simulink model "MSDRPrimaryLoop_LoadFollow"  (R2021b)
settings: Solver=VariableStepAuto  StartTime=0.0  StopTime=604900  MaxStep=1  MinStep=0.01  RelTol=1e-3
undefined symbols (not defined in the file): a_f, A_free_PHX, a_g, A_h_PHX, beta, beta_t, bubbleGeneratorArea, bubbleGeneratorDh, bubbleGeneratorElevation, bubbleGeneratorLength, bubbleGeneratorVolume, bubbleSaturationLevel, bubbleSeparatorArea, bubbleSeparatorDiameter, bubbleSeparatorDo, bubbleSeparatorLength, bubbleSeparatorSlope, bypassRatio, C0, coreFlowArea, coreFuelVolume, coreLowerPlenumArea, coreLowerPlenumHydraulicDiameter, coreLowerPlenumLength, coreLowerPlenumVolume, coreUpperPlenumArea, coreUpperPlenumHydraulicDiameter, coreUpperPlenumLength, coreUpperPlenumVolume, coreVolume, cpGraphite, dissolusionRatio, dMin, dScale, dsmConst, DXeG, Fiss_factor, fuelChannelHydrualicDiameter, fuelChannelLength, fuelDepositRatio, fuelFraction, fuelGraphiteArea, fuelGraphiteHeatTransferCoefficient, gamma0, gamma1, gamma2, generatorDsm, graphiteKDiff, graphiteUnitCellThickness, initialIodineConcentration, InitialXeMolarConcentration, InjectionRatio, injectionRatio, iodineDecayConstant, IodineDecayConstant, iodineYield, kGraphite, kScale, Lam, lam ... (+60)
libraries: fl_lib x268, nesl_utility x106, SimscapeFluids_lib x20, slpidlib x1
(part 6 of 12)

== system MSDRPrimaryLoop_LoadFollow/Pump/PumpIdeal/XenonCalcPump ==
  XeIn : Inport  OutDataTypeStr=double  Unit=kg/s
  GasRef : Inport  Port=2
  Absolute Reference (TL) : fl_lib/Thermal Liquid/Elements/Absolute Reference (TL)
      settings: SourceProductBaseCode=SS
  Demux : Demux  Outputs=2
  Gas : Subsystem
      settings: PortSchema="{\"entries\":[{\"content\":{\"sides\":[{\"content\":{\"connectorIds\":[\"In1\"]},\"type\":\"ConnectorPlacement.EquallySpacedRectSide\",\"uuid\":\"9457d014-8c8c-4ede-953a-dad1b8fcff2e\"},{\"content\":{\"connectorIds\":[\"Out1\"],\"side\":\"RIGHT\"},\"type\":\"ConnectorPlacement.EquallySpacedRectSide\",\"uuid\":\"6b13e550-1648-4662-a58b-f6f49b8dfc45\"},{\"content\":{\"connectorIds\":[\"Out2\",\"In2\"],\"side\":\"TOP\"},\"type\":\"ConnectorPlacement.EquallySpacedRectSide\",\"uuid\":\"73a4211d-b4c2-4f72-9c26-6ee46c1777bd\"},{\"content\":{\"connectorIds\":[\"In3\",\"In4\"],\"side\":\"BOTTOM\"},\"type\":\"ConnectorPlacement.EquallySpacedRectSide\",\"uuid\":\"ca62b0cd-46c8-418f-9a8b-9558726bf444\"}]},\"type\":\"ConnectorPlacement.EquallySpacedConnector\",\"uuid\":\"020f2da1-56fe-4a8a-8a2d-2f75d9123e14\"}],\"packageUris\":[\"http://schema.mathworks.com/mf0/Connector/R2020b\"],\"version\":\"1.0\"}"
  InterphaseTranfser : Subsystem
      settings: PortSchema="{\"entries\":[{\"content\":{\"sides\":[{\"content\":{\"connectorIds\":[\"In1\",\"In2\",\"In3\"]},\"type\":\"ConnectorPlacement.EquallySpacedRectSide\",\"uuid\":\"d6303689-138e-451a-a3c3-60d601b4795c\"},{\"content\":{\"connectorIds\":[\"Out1\"],\"side\":\"RIGHT\"},\"type\":\"ConnectorPlacement.EquallySpacedRectSide\",\"uuid\":\"e99266db-1ad9-4248-a3a9-dc80edd4cbf2\"},{\"content\":{\"connectorIds\":[\"LConn1\"],\"side\":\"TOP\"},\"type\":\"ConnectorPlacement.EquallySpacedRectSide\",\"uuid\":\"07679a3e-e535-452f-8d16-cac9376cf8bb\"}]},\"type\":\"ConnectorPlacement.EquallySpacedConnector\",\"uuid\":\"2a8870ca-366d-4312-85a0-e0a2095078d0\"}],\"packageUris\":[\"http://schema.mathworks.com/mf0/Connector/R2020b\"],\"version\":\"1.0\"}"
  Mux : Mux  Inputs=2
  PS Abs : fl_lib/Physical Signals/Nonlinear Operators/PS Abs
      settings: SourceProductBaseCode=SS  InternalSimscapePortConfiguration="{\"Bottom\":[],\"Left\":[{\"id\":\"I\",\"label\":\"\",\"type\":\"input\"}],\"Right\":[{\"id\":\"O\",\"label\":\"\",\"type\":\"output\"}],\"Top\":[]}"
  PS-Simulink Converter : nesl_utility/PS-Simulink Converter  PhysicalDomain=network_engine_domain  SubClassName=ps_output  LeftPortType=input  RightPortType=output  PseudoPeriodic=off  Frequencies=[]  Unit=inherit  AffineConversion=off
      settings: SourceProductBaseCode=PW,SS
  PS-Simulink Converter1 : nesl_utility/PS-Simulink Converter  PhysicalDomain=network_engine_domain  SubClassName=ps_output  LeftPortType=input  RightPortType=output  PseudoPeriodic=off  Frequencies=[]  Unit=inherit  AffineConversion=off
      settings: SourceProductBaseCode=PW,SS
  Pressure & Temperature Sensor (TL) : fl_lib/Thermal Liquid/Sensors/Pressure & Temperature Sensor (TL)
      settings: SourceProductBaseCode=SS  InternalSimscapePortConfiguration="{\"Bottom\":[],\"Left\":[{\"id\":\"A\",\"label\":\"A\",\"type\":\"foundation.thermal_liquid.thermal_liquid\"}],\"Right\":[{\"id\":\"B\",\"label\":\"B\",\"type\":\"foundation.thermal_liquid.thermal_liquid\"},{\"id\":\"P\",\"label\":\"P\",\"type\":\"output\"},{\"id\":\"T\",\"label\":\"T\",\"type\":\"output\"}],\"Top\":[]}"
  Salt : Subsystem
      settings: PortSchema="{\"entries\":[{\"content\":{\"sides\":[{\"content\":{\"connectorIds\":[\"In1\",\"In2\",\"In3\"]},\"type\":\"ConnectorPlacement.EquallySpacedRectSide\",\"uuid\":\"9457d014-8c8c-4ede-953a-dad1b8fcff2e\"},{\"content\":{\"connectorIds\":[\"Out1\"],\"side\":\"RIGHT\"},\"type\":\"ConnectorPlacement.EquallySpacedRectSide\",\"uuid\":\"6b13e550-1648-4662-a58b-f6f49b8dfc45\"},{\"content\":{\"connectorIds\":[\"In4\",\"In5\"],\"side\":\"TOP\"},\"type\":\"ConnectorPlacement.EquallySpacedRectSide\",\"uuid\":\"73a4211d-b4c2-4f72-9c26-6ee46c1777bd\"},{\"content\":{\"connectorIds\":[\"Out2\",\"In6\"],\"side\":\"BOTTOM\"},\"type\":\"ConnectorPlacement.EquallySpacedRectSide\",\"uuid\":\"ca62b0cd-46c8-418f-9a8b-9558726bf444\"}]},\"type\":\"ConnectorPlacement.EquallySpacedConnector\",\"uuid\":\"020f2da1-56fe-4a8a-8a2d-2f75d9123e14\"}],\"packageUris\":[\"http://schema.mathworks.com/mf0/Connector/R2020b\"],\"version\":\"1.0\"}"
  Volumetric Flow Rate Sensor (TL) : fl_lib/Thermal Liquid/Sensors/Volumetric Flow Rate Sensor (TL)
      settings: SourceProductBaseCode=SS  InternalSimscapePortConfiguration="{\"Bottom\":[],\"Left\":[{\"id\":\"A\",\"label\":\"A\",\"type\":\"foundation.thermal_liquid.thermal_liquid\"}],\"Right\":[{\"id\":\"B\",\"label\":\"B\",\"type\":\"foundation.thermal_liquid.thermal_liquid\"},{\"id\":\"V\",\"label\":\"V\",\"type\":\"output\"}],\"Top\":[]}"
  Inlet : PMIOPort  Side=Left
  Outlet : PMIOPort  Port=2  Side=Right
  XeOut : Outport
  wires:
  XeIn/1 -> Demux/1
  PS-Simulink Converter/1 -> Gas/4(VolumeRate), Salt/5(VolumeRate)
  GasRef/1 -> Gas/3(GasRef), InterphaseTranfser/2(GasRef), Salt/4(GasRef)
  Demux/1 -> Salt/1(XeLIn)
  [IodineSNDensity] -> Salt/2(IodineSNumberDensity)
  Demux/2 -> Gas/1(XeGIn)
  Salt/1(XeLOut) -> Mux/1
  Gas/1(XeGOut) -> Mux/2
  Mux/1 -> XeOut/1
  Salt/2(CxSalt) -> InterphaseTranfser/1(CxSalt)
  Gas/2(CxGas) -> InterphaseTranfser/3(CxGas)
  InterphaseTranfser/1(TranfserRate) -> Gas/2(Interphase), Salt/6(Interphase)
  PS-Simulink Converter1/1 -> Salt/3(T_f_ave)
  connections:
  Outlet/RConn1 -- Volumetric Flow Rate Sensor (TL)/RConn1 -- InterphaseTranfser/LConn1
  Volumetric Flow Rate Sensor (TL)/LConn1 -- Pressure & Temperature Sensor (TL)/LConn1 -- Inlet/RConn1
  Volumetric Flow Rate Sensor (TL)/RConn2 -- PS Abs/LConn1
  PS Abs/RConn1 -- PS-Simulink Converter/LConn1
  Pressure & Temperature Sensor (TL)/RConn1 -- Absolute Reference (TL)/LConn1
  Pressure & Temperature Sensor (TL)/RConn3 -- PS-Simulink Converter1/LConn1

== system MSDRPrimaryLoop_LoadFollow/Pump/PumpPysical/GasCalc ==
  GasIn : Inport
  Add : Sum  Inputs=+-
  GasExpansion : Subsystem  ReferencedSubsystem=GasExpansion
      settings: PortSchema="{\"entries\":[{\"content\":{\"sides\":[{\"content\":{\"connectorIds\":[\"LConn1\",\"In1\"]},\"type\":\"ConnectorPlacement.EquallySpacedRectSide\",\"uuid\":\"50c89675-cb8a-4964-af62-cb2014507b1d\"},{\"content\":{\"connectorIds\":[\"RConn1\",\"Out1\"],\"side\":\"RIGHT\"},\"type\":\"ConnectorPlacement.EquallySpacedRectSide\",\"uuid\":\"6b3adc78-0be5-4682-9da0-6fd41ffc4e71\"},{\"content\":{\"connectorIds\":[],\"side\":\"TOP\"},\"type\":\"ConnectorPlacement.EquallySpacedRectSide\",\"uuid\":\"5158b46f-a496-48e4-90d6-6c6dcc9e237b\"}]},\"type\":\"ConnectorPlacement.EquallySpacedConnector\",\"uuid\":\"7ff0188e-dc19-44a0-a8cf-bde33949414f\"}],\"packageUris\":[\"http://schema.mathworks.com/mf0/Connector/R2020b\"],\"version\":\"1.0\"}"
  Integrator : Integrator  InitialCondition=InjectionRatio*PumpVolume
  PS-Simulink Converter : nesl_utility/PS-Simulink Converter  PhysicalDomain=network_engine_domain  SubClassName=ps_output  LeftPortType=input  RightPortType=output  PseudoPeriodic=off  Frequencies=[]  Unit=inherit  AffineConversion=off
      settings: SourceProductBaseCode=PW,SS
  Product : Product
  VolumeToVoid : Gain  Gain=1/PumpVolume
  Ref1 : PMIOPort  Side=Left
  VolumeRate : PMIOPort  Port=2  Side=Left
  Ref2 : PMIOPort  Port=3  Side=Left
  GasOut : Outport
  wires:
  VolumeToVoid/1 -> GasExpansion/1, Add/2
  Integrator/1 -> VolumeToVoid/1
  GasIn/1 -> Add/1
  Add/1 -> Product/1
  Product/1 -> Integrator/1
  PS-Simulink Converter/1 -> Product/2
  GasExpansion/1 -> GasOut/1
  connections:
  PS-Simulink Converter/LConn1 -- VolumeRate/RConn1
  GasExpansion/LConn1 -- Ref1/RConn1
  GasExpansion/RConn1 -- Ref2/RConn1

== system MSDRPrimaryLoop_LoadFollow/Pump/PumpPysical/PumpPhysics&Control ==
  note: Pump capacity is linearly scaled to 3 times of the deisgn, as only one loop is modeled.
  GasRef : Inport
  2PModification : Subsystem  ReferencedSubsystem=TwoPhaseModification
      settings: PortSchema="{\"entries\":[{\"content\":{\"sides\":[{\"content\":{\"connectorIds\":[\"LConn1\"]},\"type\":\"ConnectorPlacement.EquallySpacedRectSide\",\"uuid\":\"7546b4b7-b669-49c8-8f27-f696391ea3ad\"},{\"content\":{\"connectorIds\":[\"RConn1\"],\"side\":\"RIGHT\"},\"type\":\"ConnectorPlacement.EquallySpacedRectSide\",\"uuid\":\"0e6176f2-177c-4327-bcfa-9a190fe9083f\"},{\"content\":{\"connectorIds\":[\"RConn2\"],\"side\":\"TOP\"},\"type\":\"ConnectorPlacement.EquallySpacedRectSide\",\"uuid\":\"16faf74c-4635-4009-a5b3-33dd03b625c6\"},{\"content\":{\"connectorIds\":[\"LConn2\",\"In1\"],\"side\":\"BOTTOM\"},\"type\":\"ConnectorPlacement.EquallySpacedRectSide\",\"uuid\":\"2081d73b-bb08-4ad9-b5c8-e48a4e9c4e20\"}]},\"type\":\"ConnectorPlacement.EquallySpacedConnector\",\"uuid\":\"243e4075-206b-4747-a8bc-b8f10d9a577f\"}],\"packageUris\":[\"http://schema.mathworks.com/mf0/Connector/R2020b\"],\"version\":\"1.0\"}"
  Centrifugal Pump (TL) : SimscapeFluids_lib/Thermal Liquid/Pumps & Motors/Centrifugal Pump (TL)  pump_parameterization=fluids.thermal_liquid.pumps_motors.enum.CentrifugalPumpParameterization.Nominal  capacity_ref_nominal=v_dot m^3/s  head_ref_nominal=45.7200 m  power_ref_nominal=0.85 kW  head_ref_max=70 m  capacity_ref_max=v_dot*2 m^3/s  omega_ref_analytic=2500 rpm  flow_rate_1D_TLU=[16.67, 30, 40, 53.33, 66.67, 83.33] lpm  head_1D_TLU=[50, 47.5, 45, 40, 35, 25] m  power_1D_TLU=[.6, .75, .85, .93, .98, .99] kW  omega_ref_1D=3500 rpm  rho_ref_1D=998.21 kg/m^3  flow_rate_2D_TLU=[16.67, 23.33, 30, 40, 53.33, 60] lpm  omega_2D_TLU=[2450, 2800, 3150, 3500] rpm  head_2D_TLU=[25, 32.7, 42.5, 50; 24, 31.7, 41, 49; 22.7, 30.5, 39, 47.5; 20, 28, 36, 45; 15.7, 24, 32, 40; 12.5, 21, 29.5, 37.5] m  power_2D_TLU=[.28, .38, .5, .6; .31, .41, .55, .68; .33, .44, .6, .75; .36, .48, .65, .83; .38, .53, .72, .93; .39, .55, .75, .97] kW  rho_ref_2D=998.21 kg/m^3  diameter_ratio=1  mech_orientation=fluids.thermal_liquid.pumps_motors.enum.CentrifugalPumpMechOrientation.Positive  area=0.25*pi*Pipe1Diameter^2*3 m^2
      settings: SourceProductBaseCode=SH  LogSimulationData=on  InternalSimscapePortConfiguration="{\"Bottom\":[],\"Left\":[{\"id\":\"A\",\"label\":\"A\",\"type\":\"foundation.thermal_liquid.thermal_liquid\"},{\"id\":\"B\",\"label\":\"B\",\"type\":\"foundation.thermal_liquid.thermal_liquid\"}],\"Right\":[{\"id\":\"R\",\"label\":\"R\",\"type\":\"foundation.mechanical.rotational.rotational\"},{\"id\":\"C\",\"label\":\"C\",\"type\":\"foundation.mechanical.rotational.rotational\"}],\"Top\":[]}"
  Ideal Angular Velocity Source : fl_lib/Mechanical/Mechanical Sources/Ideal Angular Velocity Source
  Mechanical Rotational Reference1 : fl_lib/Mechanical/Rotational Elements/Mechanical Rotational Reference
  Mechanical Rotational Reference2 : fl_lib/Mechanical/Rotational Elements/Mechanical Rotational Reference
  PS Abs : fl_lib/Physical Signals/Nonlinear Operators/PS Abs
      settings: SourceProductBaseCode=SS  InternalSimscapePortConfiguration="{\"Bottom\":[],\"Left\":[{\"id\":\"I\",\"label\":\"\",\"type\":\"input\"}],\"Right\":[{\"id\":\"O\",\"label\":\"\",\"type\":\"output\"}],\"Top\":[]}"
  Pump Drive Control : Subsystem
      settings: PortSchema="{\"entries\":[{\"content\":{\"sides\":[{\"content\":{\"connectorIds\":[\"LConn1\"]},\"type\":\"ConnectorPlacement.EquallySpacedRectSide\",\"uuid\":\"e4f8502b-306b-4a14-917e-1e63d742dab0\"},{\"content\":{\"connectorIds\":[\"RConn1\"],\"side\":\"RIGHT\"},\"type\":\"ConnectorPlacement.EquallySpacedRectSide\",\"uuid\":\"711ed699-17a5-44fb-968d-5c6132c14151\"},{\"content\":{\"connectorIds\":[\"LConn2\"],\"side\":\"TOP\"},\"type\":\"ConnectorPlacement.EquallySpacedRectSide\",\"uuid\":\"4e78022b-898e-4d83-b0bd-b0ef3bc93923\"},{\"content\":{\"connectorIds\":[],\"side\":\"BOTTOM\"},\"type\":\"ConnectorPlacement.EquallySpacedRectSide\",\"uuid\":\"a73c464e-7373-4480-b96b-ebe915c98bdf\"}]},\"type\":\"ConnectorPlacement.EquallySpacedConnector\",\"uuid\":\"08f647c4-2347-4031-ac16-01138a2dbc22\"}],\"packageUris\":[\"http://schema.mathworks.com/mf0/Connector/R2020b\"],\"version\":\"1.0\"}"
  PumpBowl : fl_lib/Thermal Liquid/Elements/Reservoir (TL)  pressure_spec=foundation.enum.pressure_spec.specified  reservoir_pressure=P0 Pa  reservoir_temperature=700 K  area=0.01 m^2
      settings: SourceProductBaseCode=SS  LogSimulationData=on
  Volumetric Flow Rate Sensor (TL) : fl_lib/Thermal Liquid/Sensors/Volumetric Flow Rate Sensor (TL)
      settings: SourceProductBaseCode=SS  InternalSimscapePortConfiguration="{\"Bottom\":[],\"Left\":[{\"id\":\"A\",\"label\":\"A\",\"type\":\"foundation.thermal_liquid.thermal_liquid\"}],\"Right\":[{\"id\":\"B\",\"label\":\"B\",\"type\":\"foundation.thermal_liquid.thermal_liquid\"},{\"id\":\"V\",\"label\":\"V\",\"type\":\"output\"}],\"Top\":[]}"
  Inlet : PMIOPort  Side=Left
  Outlet : PMIOPort  Port=2  Side=Right
  VolumeRate : PMIOPort  Port=3  Side=Right
  wires:
  GasRef/1 -> 2PModification/1
  connections:
  Ideal Angular Velocity Source/RConn1 -- Pump Drive Control/LConn1
  Centrifugal Pump (TL)/LConn1 -- 2PModification/LConn2 -- PumpBowl/LConn1 -- Inlet/RConn1 -- Pump Drive Control/RConn1
  Centrifugal Pump (TL)/RConn1 -- Ideal Angular Velocity Source/LConn1
  Centrifugal Pump (TL)/RConn2 -- Mechanical Rotational Reference2/LConn1
  Ideal Angular Velocity Source/RConn2 -- Mechanical Rotational Reference1/LConn1
  Volumetric Flow Rate Sensor (TL)/RConn2 -- PS Abs/LConn1
  Centrifugal Pump (TL)/LConn2 -- Volumetric Flow Rate Sensor (TL)/LConn1
  PS Abs/RConn1 -- VolumeRate/RConn1 -- Pump Drive Control/LConn2
  Volumetric Flow Rate Sensor (TL)/RConn1 -- 2PModification/RConn2 -- 2PModification/LConn1
  2PModification/RConn1 -- Outlet/RConn1

== system MSDRPrimaryLoop_LoadFollow/Pump/PumpPysical/XenonCalc ==
  XeIn : Inport
  Add : Sum  Inputs=|+--
  Decay : Gain  Gain=XeDecayConstant
  MassToConc : Gain  Gain=1/PumpVolume
  PS-Simulink Converter : nesl_utility/PS-Simulink Converter  PhysicalDomain=network_engine_domain  SubClassName=ps_output  LeftPortType=input  RightPortType=output  PseudoPeriodic=off  Frequencies=[]  Unit=inherit  AffineConversion=off
      settings: SourceProductBaseCode=PW,SS
  Product : Product
  TotalMass : Integrator  InitialCondition=InitialXeMolarConcentration*PumpVolume*0.135
  VolumeRate : PMIOPort  Side=Left
  XeOut : Outport
  wires:
  Add/1 -> TotalMass/1
  XeIn/1 -> Add/1
  Product/1 -> Add/3, XeOut/1
  TotalMass/1 -> Decay/1, MassToConc/1
  PS-Simulink Converter/1 -> Product/1
  MassToConc/1 -> Product/2
  Decay/1 -> Add/2
  connections:
  VolumeRate/RConn1 -- PS-Simulink Converter/LConn1

== system MSDRPrimaryLoop_LoadFollow/Reactor/CoreTH&Inerti/Core ==
  XeIn : Inport
  GasIn : Inport  Port=2
  IodineSNumberDensity : Inport  Port=3
  NeutronFraction : Inport  Port=4
  DecayFraction : Inport  Port=5
  CoreTH : Subsystem  mask{N_nodes=4, FuelDepositRatio=fuelDepositRatio, k_graphite=kGraphite, cp_graphite=cpGraphite, rho_graphite=rhoGraphite, UnitCellGraphiteThickness=graphiteUnitCellThickness, h_fg=fuelGraphiteHeatTransferCoefficient, T0=T0, P0=P0}
      mask prompts: N_nodes "Number Of Nodes"; k_graphite "Graphite Thermal Conductivity"; cp_graphite "Graphite Specific Thermal Capacity"; rho_graphite "Graphite Density"; UnitCellGraphiteThickness "Unit Cell Graphite Thickness"; h_fg "Fuel Graphite Heat Transfer Coefficient"; T0 "Initial Temperature"; P0 "Initial Pressure"
      settings: PortSchema="{\"entries\":[{\"content\":{\"sides\":[{\"content\":{\"connectorIds\":[\"LConn1\",\"LConn2\",\"LConn3\"]},\"type\":\"ConnectorPlacement.EquallySpacedRectSide\",\"uuid\":\"1c20b62e-1aca-4cc3-9434-4d9ffc0779e4\"},{\"content\":{\"connectorIds\":[\"Out1\",\"RConn1\"],\"side\":\"RIGHT\"},\"type\":\"ConnectorPlacement.EquallySpacedRectSide\",\"uuid\":\"cbe92cdf-09f7-4580-a6a7-168080192112\"},{\"content\":{\"connectorIds\":[\"In1\",\"In2\"],\"side\":\"TOP\"},\"type\":\"ConnectorPlacement.EquallySpacedRectSide\",\"uuid\":\"70a4d7aa-1432-4349-89f0-42a0194e580f\"},{\"content\":{\"connectorIds\":[\"In3\"],\"side\":\"BOTTOM\"},\"type\":\"ConnectorPlacement.EquallySpacedRectSide\",\"uuid\":\"7c92aed1-92dd-461a-937a-8dd840527e94\"}]},\"type\":\"ConnectorPlacement.EquallySpacedConnector\",\"uuid\":\"1a67b279-14f5-41a4-8cd2-abe76a0f00c3\"}],\"packageUris\":[\"http://schema.mathworks.com/mf0/Connector/R2020b\"],\"version\":\"1.0\"}"
  CoreXenonCalc : Subsystem
      settings: PortSchema="{\"entries\":[{\"content\":{\"sides\":[{\"content\":{\"connectorIds\":[\"In1\",\"LConn1\"]},\"type\":\"ConnectorPlacement.EquallySpacedRectSide\",\"uuid\":\"82f8e7e7-fd89-4597-952e-64db268d0190\"},{\"content\":{\"connectorIds\":[\"Out1\",\"Out2\",\"RConn1\"],\"side\":\"RIGHT\"},\"type\":\"ConnectorPlacement.EquallySpacedRectSide\",\"uuid\":\"4b3edad1-18f8-43fa-96ee-a24bb3384b59\"},{\"content\":{\"connectorIds\":[\"In2\",\"In3\",\"In4\"],\"side\":\"TOP\"},\"type\":\"ConnectorPlacement.EquallySpacedRectSide\",\"uuid\":\"43d4f51d-f841-40d6-804e-7f238a90dabe\"},{\"content\":{\"connectorIds\":[\"In5\",\"In6\"],\"side\":\"BOTTOM\"},\"type\":\"ConnectorPlacement.EquallySpacedRectSide\",\"uuid\":\"350f2274-4108-4e6e-a637-0ae7118de3f0\"}]},\"type\":\"ConnectorPlacement.EquallySpacedConnector\",\"uuid\":\"d7e795ea-9d5d-4a8c-83ab-dab42197cc2f\"}],\"packageUris\":[\"http://schema.mathworks.com/mf0/Connector/R2020b\"],\"version\":\"1.0\"}"
  Delay One Step : Delay  DelayLength=1  InitialCondition=T0
  PLossFunc : Subsystem
      settings: PortSchema="{\"entries\":[{\"content\":{\"sides\":[{\"content\":{\"connectorIds\":[\"Out1\",\"LConn1\"]},\"type\":\"ConnectorPlacement.EquallySpacedRectSide\",\"uuid\":\"95ca4545-c473-4e31-844b-c43557042c16\"},{\"content\":{\"connectorIds\":[\"RConn1\"],\"side\":\"RIGHT\"},\"type\":\"ConnectorPlacement.EquallySpacedRectSide\",\"uuid\":\"f9304c30-8684-4a05-a34b-3121610e628d\"},{\"content\":{\"connectorIds\":[],\"side\":\"TOP\"},\"type\":\"ConnectorPlacement.EquallySpacedRectSide\",\"uuid\":\"64c7a4d8-8539-4303-ae81-4015bd1451af\"}]},\"type\":\"ConnectorPlacement.EquallySpacedConnector\",\"uuid\":\"40c12b2f-fb9d-4a19-b6f1-e93ae1fd4d68\"}],\"packageUris\":[\"http://schema.mathworks.com/mf0/Connector/R2020b\"],\"version\":\"1.0\"}"
  SolubilityReduction : Subsystem
      settings: PortSchema="{\"entries\":[{\"content\":{\"sides\":[{\"content\":{\"connectorIds\":[\"In1\",\"In2\"]},\"type\":\"ConnectorPlacement.EquallySpacedRectSide\",\"uuid\":\"faacc406-4069-496b-af99-41d2aed9dfc2\"},{\"content\":{\"connectorIds\":[\"Out1\",\"Out2\",\"Out3\"],\"side\":\"RIGHT\"},\"type\":\"ConnectorPlacement.EquallySpacedRectSide\",\"uuid\":\"94f1539c-5515-4bd6-bffb-3a5caf43f7b6\"},{\"content\":{\"connectorIds\":[],\"side\":\"TOP\"},\"type\":\"ConnectorPlacement.EquallySpacedRectSide\",\"uuid\":\"d17dce47-2058-4206-8706-4dc771d04045\"},{\"content\":{\"connectorIds\":[\"Out4\"],\"side\":\"BOTTOM\"},\"type\":\"ConnectorPlacement.EquallySpacedRectSide\",\"uuid\":\"97529780-84fa-4776-a404-e5a3e7258a40\"}]},\"type\":\"ConnectorPlacement.EquallySpacedConnector\",\"uuid\":\"1ce9374c-8c3e-43ec-9da7-5b483b5e3d48\"}],\"packageUris\":[\"http://schema.mathworks.com/mf0/Connector/R2020b\"],\"version\":\"1.0\"}"
  Subsystem : Subsystem
  Subsystem1 : Subsystem
      settings: PortSchema="{\"entries\":[{\"content\":{\"sides\":[{\"content\":{\"connectorIds\":[\"In1\",\"In2\"]},\"type\":\"ConnectorPlacement.EquallySpacedRectSide\",\"uuid\":\"2a068eb5-92e4-43e3-b748-0f561ebb2f0e\"},{\"content\":{\"connectorIds\":[\"Out1\",\"Out2\"],\"side\":\"RIGHT\"},\"type\":\"ConnectorPlacement.EquallySpacedRectSide\",\"uuid\":\"d07e14f8-d0ba-4d92-9a78-613216e777c8\"},{\"content\":{\"connectorIds\":[\"LConn1\",\"LConn2\",\"Out3\",\"LConn3\"],\"side\":\"TOP\"},\"type\":\"ConnectorPlacement.EquallySpacedRectSide\",\"uuid\":\"40c9f9fd-9b75-4721-9a62-c538b0ea8b4c\"}]},\"type\":\"ConnectorPlacement.EquallySpacedConnector\",\"uuid\":\"1283fec4-e55b-4051-bba7-bc8dde4dc12d\"}],\"packageUris\":[\"http://schema.mathworks.com/mf0/Connector/R2020b\"],\"version\":\"1.0\"}"
  Subsystem2 : Subsystem  Variant=on  VariantControlMode=label  VariantControl=Choice  LabelModeActiveChoice=Constant
      settings: PortSchema="{\"entries\":[{\"content\":{\"sides\":[{\"content\":{\"connectorIds\":[\"In1\",\"In2\",\"In3\"]},\"type\":\"ConnectorPlacement.EquallySpacedRectSide\",\"uuid\":\"cfe1ce7c-1611-431e-9412-2b3caba343b3\"},{\"content\":{\"connectorIds\":[\"Out1\",\"Out2\"],\"side\":\"RIGHT\"},\"type\":\"ConnectorPlacement.EquallySpacedRectSide\",\"uuid\":\"0c689a27-e89a-4b17-8ea0-ad5769387ae3\"},{\"content\":{\"connectorIds\":[\"In4\"],\"side\":\"TOP\"},\"type\":\"ConnectorPlacement.EquallySpacedRectSide\",\"uuid\":\"a650924a-5c90-44bf-97de-77f017d49b56\"},{\"content\":{\"connectorIds\":[\"In5\"],\"side\":\"BOTTOM\"},\"type\":\"ConnectorPlacement.EquallySpacedRectSide\",\"uuid\":\"af91b143-b368-4d0c-8cc7-2ed084fb2df7\"}]},\"type\":\"ConnectorPlacement.EquallySpacedConnector\",\"uuid\":\"a7e506ef-3f33-4307-859c-c22ba4b969e5\"}],\"packageUris\":[\"http://schema.mathworks.com/mf0/Connector/R2020b\"],\"version\":\"1.0\"}"
  Volumetric Flow Rate Sensor (TL) : fl_lib/Thermal Liquid/Sensors/Volumetric Flow Rate Sensor (TL)
      settings: SourceProductBaseCode=SS  InternalSimscapePortConfiguration="{\"Bottom\":[],\"Left\":[{\"id\":\"A\",\"label\":\"A\",\"type\":\"foundation.thermal_liquid.thermal_liquid\"}],\"Right\":[{\"id\":\"B\",\"label\":\"B\",\"type\":\"foundation.thermal_liquid.thermal_liquid\"},{\"id\":\"V\",\"label\":\"V\",\"type\":\"output\"}],\"Top\":[]}"
  Inlet : PMIOPort  Side=Left
  InletSideHeatTranfser : PMIOPort  Port=2  Side=Left
  Outlet : PMIOPort  Port=3  Side=Right
  " Outlet Side Heat Transfer" : PMIOPort  Port=4  Side=Right
  XeOut : Outport
  GasOut : Outport  Port=2
  "TotalXeCrossSection, [cm^2]" : Outport  Port=3
  Temperatures : Outport  Port=4
  wires:
  NeutronFraction/1 -> CoreTH/2(NeutronFraction), CoreXenonCalc/4(NeutronFraction)
  CoreTH/1(Temperatures) -> Temperatures/1, Subsystem/1(Temperatures)
  XeIn/1 -> SolubilityReduction/1(XeIn)
  Delay One Step/1 -> CoreXenonCalc/3(T_f_ave), Subsystem2/4(Temperature)
  CoreXenonCalc/2("TotalXeCrossSection, [cm^2]") -> "TotalXeCrossSection, [cm^2]"/1
  Subsystem/1(T_f_ave) -> Delay One Step/1
  IodineSNumberDensity/1 -> CoreXenonCalc/2(IodineSNumberDensity)
  SolubilityReduction/1(XeOut) -> CoreXenonCalc/1(XeIn)
  GasIn/1 -> SolubilityReduction/2(GasIn)
  DecayFraction/1 -> CoreTH/1(DecayFraction)
  Subsystem1/3(GasRefOut) -> CoreTH/3(GasRef), CoreXenonCalc/6(GasRef)
  SolubilityReduction/2(GasOut) -> Subsystem1/1(GasIn)
  SolubilityReduction/3(AbsorbedGas) -> Subsystem1/2(Absorbed)
  PLossFunc/1(PLoss) -> CoreXenonCalc/5(PLoss)
  CoreXenonCalc/1(XeOut) -> Subsystem2/1(XeIn)
  Subsystem1/1(GasOut) -> Subsystem2/2(GasIn)
  Subsystem1/2(AbsorbedOut) -> Subsystem2/3(AbsorbedOut)
  SolubilityReduction/4(ModeSwitch) -> Subsystem2/5(ModeSwitch)
  Subsystem2/1(GasOut) -> GasOut/1
  Subsystem2/2(XeOut) -> XeOut/1
  connections:
  Volumetric Flow Rate Sensor (TL)/LConn1 -- PLossFunc/LConn1 -- Subsystem1/LConn1 -- Inlet/RConn1
  Volumetric Flow Rate Sensor (TL)/RConn1 -- CoreXenonCalc/LConn1
  CoreXenonCalc/RConn1 -- CoreTH/LConn1
  CoreTH/RConn1 -- Outlet/RConn1 -- PLossFunc/RConn1 -- Subsystem1/LConn3
  Volumetric Flow Rate Sensor (TL)/RConn2 -- Subsystem1/LConn2
  CoreTH/LConn2 -- InletSideHeatTranfser/RConn1
  CoreTH/LConn3 -- " Outlet Side Heat Transfer"/RConn1

== system MSDRPrimaryLoop_LoadFollow/Reactor/CoreTH&Inerti/LowerPlenum ==
  XeIn : Inport
  GasIn : Inport  Port=2
  Add : Sum  Inputs=|++
  Delay One Step : Delay  DelayLength=1
  Gain : Gain  Gain=0.5
  GasCalc : Subsystem  mask{Volume=Volume}
      settings: PortSchema="{\"entries\":[{\"content\":{\"sides\":[{\"content\":{\"connectorIds\":[\"In1\"]},\"type\":\"ConnectorPlacement.EquallySpacedRectSide\",\"uuid\":\"a8e1ce06-71c9-462d-8d5c-7a3e078b5544\"},{\"content\":{\"connectorIds\":[\"Out1\"],\"side\":\"RIGHT\"},\"type\":\"ConnectorPlacement.EquallySpacedRectSide\",\"uuid\":\"2c63a1ce-15e2-4b17-a432-f9f40781bd58\"},{\"content\":{\"connectorIds\":[\"LConn1\",\"LConn2\",\"LConn3\"],\"side\":\"TOP\"},\"type\":\"ConnectorPlacement.EquallySpacedRectSide\",\"uuid\":\"abc20e07-15eb-475f-be7f-cc96378523a1\"},{\"content\":{\"connectorIds\":[],\"side\":\"BOTTOM\"},\"type\":\"ConnectorPlacement.EquallySpacedRectSide\",\"uuid\":\"ab58f362-f4c2-4e86-bda0-802426066295\"}]},\"type\":\"ConnectorPlacement.EquallySpacedConnector\",\"uuid\":\"b54d49a9-048b-4912-bf18-92a7ef5e8aff\"}],\"packageUris\":[\"http://schema.mathworks.com/mf0/Connector/R2020b\"],\"version\":\"1.0\"}"
  LowerPlenum : Subsystem
      settings: PortSchema="{\"entries\":[{\"content\":{\"sides\":[{\"content\":{\"connectorIds\":[\"LConn1\",\"In1\"]},\"type\":\"ConnectorPlacement.EquallySpacedRectSide\",\"uuid\":\"0f255306-ec83-4423-ac41-a2708bd1ec44\"},{\"content\":{\"connectorIds\":[\"RConn1\",\"RConn2\"],\"side\":\"RIGHT\"},\"type\":\"ConnectorPlacement.EquallySpacedRectSide\",\"uuid\":\"650fb4ea-7b32-4c45-8538-9785d9ca64bf\"},{\"content\":{\"connectorIds\":[],\"side\":\"TOP\"},\"type\":\"ConnectorPlacement.EquallySpacedRectSide\",\"uuid\":\"434d3568-54a4-4787-a287-69f15ef478cb\"},{\"content\":{\"connectorIds\":[\"RConn3\"],\"side\":\"BOTTOM\"},\"type\":\"ConnectorPlacement.EquallySpacedRectSide\",\"uuid\":\"5b0b510d-1175-4508-bbe9-65b563e28484\"}]},\"type\":\"ConnectorPlacement.EquallySpacedConnector\",\"uuid\":\"b18d9c84-3d71-444b-a89d-79c3dc70d4d9\"}],\"packageUris\":[\"http://schema.mathworks.com/mf0/Connector/R2020b\"],\"version\":\"1.0\"}"
  PLossFunc : Subsystem
      settings: PortSchema="{\"entries\":[{\"content\":{\"sides\":[{\"content\":{\"connectorIds\":[\"Out1\",\"LConn1\"]},\"type\":\"ConnectorPlacement.EquallySpacedRectSide\",\"uuid\":\"95ca4545-c473-4e31-844b-c43557042c16\"},{\"content\":{\"connectorIds\":[\"RConn1\"],\"side\":\"RIGHT\"},\"type\":\"ConnectorPlacement.EquallySpacedRectSide\",\"uuid\":\"f9304c30-8684-4a05-a34b-3121610e628d\"},{\"content\":{\"connectorIds\":[],\"side\":\"TOP\"},\"type\":\"ConnectorPlacement.EquallySpacedRectSide\",\"uuid\":\"64c7a4d8-8539-4303-ae81-4015bd1451af\"}]},\"type\":\"ConnectorPlacement.EquallySpacedConnector\",\"uuid\":\"40c12b2f-fb9d-4a19-b6f1-e93ae1fd4d68\"}],\"packageUris\":[\"http://schema.mathworks.com/mf0/Connector/R2020b\"],\"version\":\"1.0\"}"
  XenonCalc : Subsystem  mask{Volume=Volume, Area=Area, Length=Length, Dh=Dh, Elevation=Elevation}
      mask prompts: Dh "Hydraulic Diameter"
      settings: PortSchema="{\"entries\":[{\"content\":{\"sides\":[{\"content\":{\"connectorIds\":[\"LConn1\",\"In1\"]},\"type\":\"ConnectorPlacement.EquallySpacedRectSide\",\"uuid\":\"82f8e7e7-fd89-4597-952e-64db268d0190\"},{\"content\":{\"connectorIds\":[\"RConn1\",\"Out1\"],\"side\":\"RIGHT\"},\"type\":\"ConnectorPlacement.EquallySpacedRectSide\",\"uuid\":\"4b3edad1-18f8-43fa-96ee-a24bb3384b59\"},{\"content\":{\"connectorIds\":[\"In2\"],\"side\":\"TOP\"},\"type\":\"ConnectorPlacement.EquallySpacedRectSide\",\"uuid\":\"43d4f51d-f841-40d6-804e-7f238a90dabe\"},{\"content\":{\"connectorIds\":[\"In3\"],\"side\":\"BOTTOM\"},\"type\":\"ConnectorPlacement.EquallySpacedRectSide\",\"uuid\":\"350f2274-4108-4e6e-a637-0ae7118de3f0\"}]},\"type\":\"ConnectorPlacement.EquallySpacedConnector\",\"uuid\":\"d7e795ea-9d5d-4a8c-83ab-dab42197cc2f\"}],\"packageUris\":[\"http://schema.mathworks.com/mf0/Connector/R2020b\"],\"version\":\"1.0\"}"
  Inlet : PMIOPort  Side=Left
  Outlet : PMIOPort  Port=2  Side=Right
  Thermal : PMIOPort  Port=3  Side=Left
  XeOut : Outport
  GasOut : Outport  Port=2
  wires:
  XenonCalc/1(XeOut) -> XeOut/1
  Add/1 -> Gain/1
  GasCalc/1(GasOut) -> GasOut/1, Add/2
  Gain/1 -> Delay One Step/1
  GasIn/1 -> GasCalc/1(GasIn), Add/1
  Delay One Step/1 -> XenonCalc/3(GasRef), LowerPlenum/1(GasInRef)
  XeIn/1 -> XenonCalc/1(XeIn)
  PLossFunc/1(PLoss) -> XenonCalc/2(PLoss)
  connections:
  Inlet/RConn1 -- GasCalc/LConn1 -- XenonCalc/LConn1
  Outlet/RConn1 -- PLossFunc/RConn1 -- GasCalc/LConn3 -- LowerPlenum/RConn2
  GasCalc/LConn2 -- LowerPlenum/RConn3
  XenonCalc/RConn1 -- PLossFunc/LConn1 -- LowerPlenum/LConn1
  LowerPlenum/RConn1 -- Thermal/RConn1

== system MSDRPrimaryLoop_LoadFollow/Reactor/CoreTH&Inerti/UpperPlenum ==
  XeIn : Inport
  GasIn : Inport  Port=2
  Add : Sum  Inputs=|++
  Delay One Step : Delay  DelayLength=1
  Gain : Gain  Gain=0.5
  GasCalc : Subsystem  mask{Volume=Volume}
      settings: PortSchema="{\"entries\":[{\"content\":{\"sides\":[{\"content\":{\"connectorIds\":[\"In1\"]},\"type\":\"ConnectorPlacement.EquallySpacedRectSide\",\"uuid\":\"a8e1ce06-71c9-462d-8d5c-7a3e078b5544\"},{\"content\":{\"connectorIds\":[\"Out1\"],\"side\":\"RIGHT\"},\"type\":\"ConnectorPlacement.EquallySpacedRectSide\",\"uuid\":\"2c63a1ce-15e2-4b17-a432-f9f40781bd58\"},{\"content\":{\"connectorIds\":[\"LConn1\",\"LConn2\",\"LConn3\"],\"side\":\"TOP\"},\"type\":\"ConnectorPlacement.EquallySpacedRectSide\",\"uuid\":\"abc20e07-15eb-475f-be7f-cc96378523a1\"},{\"content\":{\"connectorIds\":[],\"side\":\"BOTTOM\"},\"type\":\"ConnectorPlacement.EquallySpacedRectSide\",\"uuid\":\"ab58f362-f4c2-4e86-bda0-802426066295\"}]},\"type\":\"ConnectorPlacement.EquallySpacedConnector\",\"uuid\":\"b54d49a9-048b-4912-bf18-92a7ef5e8aff\"}],\"packageUris\":[\"http://schema.mathworks.com/mf0/Connector/R2020b\"],\"version\":\"1.0\"}"
  PLossFunc : Subsystem
      settings: PortSchema="{\"entries\":[{\"content\":{\"sides\":[{\"content\":{\"connectorIds\":[\"Out1\",\"LConn1\"]},\"type\":\"ConnectorPlacement.EquallySpacedRectSide\",\"uuid\":\"95ca4545-c473-4e31-844b-c43557042c16\"},{\"content\":{\"connectorIds\":[\"RConn1\"],\"side\":\"RIGHT\"},\"type\":\"ConnectorPlacement.EquallySpacedRectSide\",\"uuid\":\"f9304c30-8684-4a05-a34b-3121610e628d\"},{\"content\":{\"connectorIds\":[],\"side\":\"TOP\"},\"type\":\"ConnectorPlacement.EquallySpacedRectSide\",\"uuid\":\"64c7a4d8-8539-4303-ae81-4015bd1451af\"}]},\"type\":\"ConnectorPlacement.EquallySpacedConnector\",\"uuid\":\"40c12b2f-fb9d-4a19-b6f1-e93ae1fd4d68\"}],\"packageUris\":[\"http://schema.mathworks.com/mf0/Connector/R2020b\"],\"version\":\"1.0\"}"
  UpperPlenum : Subsystem
      settings: PortSchema="{\"entries\":[{\"content\":{\"sides\":[{\"content\":{\"connectorIds\":[\"LConn1\",\"In1\"]},\"type\":\"ConnectorPlacement.EquallySpacedRectSide\",\"uuid\":\"0f255306-ec83-4423-ac41-a2708bd1ec44\"},{\"content\":{\"connectorIds\":[\"RConn1\",\"RConn2\"],\"side\":\"RIGHT\"},\"type\":\"ConnectorPlacement.EquallySpacedRectSide\",\"uuid\":\"650fb4ea-7b32-4c45-8538-9785d9ca64bf\"},{\"content\":{\"connectorIds\":[],\"side\":\"TOP\"},\"type\":\"ConnectorPlacement.EquallySpacedRectSide\",\"uuid\":\"434d3568-54a4-4787-a287-69f15ef478cb\"},{\"content\":{\"connectorIds\":[\"RConn3\"],\"side\":\"BOTTOM\"},\"type\":\"ConnectorPlacement.EquallySpacedRectSide\",\"uuid\":\"5b0b510d-1175-4508-bbe9-65b563e28484\"}]},\"type\":\"ConnectorPlacement.EquallySpacedConnector\",\"uuid\":\"b18d9c84-3d71-444b-a89d-79c3dc70d4d9\"}],\"packageUris\":[\"http://schema.mathworks.com/mf0/Connector/R2020b\"],\"version\":\"1.0\"}"
  XenonCalc : Subsystem  mask{Volume=Volume, Area=Area, Length=Length, Dh=Dh, Elevation=Elevation}
      mask prompts: Dh "Hydraulic Diameter"
      settings: PortSchema="{\"entries\":[{\"content\":{\"sides\":[{\"content\":{\"connectorIds\":[\"LConn1\",\"In1\"]},\"type\":\"ConnectorPlacement.EquallySpacedRectSide\",\"uuid\":\"82f8e7e7-fd89-4597-952e-64db268d0190\"},{\"content\":{\"connectorIds\":[\"RConn1\",\"Out1\"],\"side\":\"RIGHT\"},\"type\":\"ConnectorPlacement.EquallySpacedRectSide\",\"uuid\":\"4b3edad1-18f8-43fa-96ee-a24bb3384b59\"},{\"content\":{\"connectorIds\":[\"In2\"],\"side\":\"TOP\"},\"type\":\"ConnectorPlacement.EquallySpacedRectSide\",\"uuid\":\"43d4f51d-f841-40d6-804e-7f238a90dabe\"},{\"content\":{\"connectorIds\":[\"In3\"],\"side\":\"BOTTOM\"},\"type\":\"ConnectorPlacement.EquallySpacedRectSide\",\"uuid\":\"350f2274-4108-4e6e-a637-0ae7118de3f0\"}]},\"type\":\"ConnectorPlacement.EquallySpacedConnector\",\"uuid\":\"d7e795ea-9d5d-4a8c-83ab-dab42197cc2f\"}],\"packageUris\":[\"http://schema.mathworks.com/mf0/Connector/R2020b\"],\"version\":\"1.0\"}"
  Inlet : PMIOPort  Side=Left
  Outlet : PMIOPort  Port=2  Side=Right
  Thermal : PMIOPort  Port=3  Side=Left
  XeOut : Outport
  GasOut : Outport  Port=2
  wires:
  XenonCalc/1(XeOut) -> XeOut/1
  Add/1 -> Gain/1
  GasCalc/1(GasOut) -> GasOut/1, Add/2
  Gain/1 -> Delay One Step/1
  GasIn/1 -> GasCalc/1(GasIn), Add/1
  Delay One Step/1 -> XenonCalc/3(GasRef), UpperPlenum/1(GasInRef)
  XeIn/1 -> XenonCalc/1(XeIn)
  PLossFunc/1(PLoss) -> XenonCalc/2(PLoss)
  connections:
  Inlet/RConn1 -- XenonCalc/LConn1 -- GasCalc/LConn1
  Outlet/RConn1 -- PLossFunc/RConn1 -- GasCalc/LConn3 -- UpperPlenum/RConn2
  GasCalc/LConn2 -- UpperPlenum/RConn3
  PLossFunc/LConn1 -- XenonCalc/RConn1 -- UpperPlenum/LConn1
  UpperPlenum/RConn1 -- Thermal/RConn1

== system MSDRPrimaryLoop_LoadFollow/Reactor/Reactivity&PKE/Ideal ==
  FlowFrac : Inport
  CORE TEMPERATURE : Inport  Port=2
  "XeCore, [cm^2]" : Inport  Port=3
  From Workspace : FromWorkspace  VariableName=powerSignal  OutputAfterFinalValue=Holding final value
  Product : Product
  Step : Step  Time=100  Before=0.001  After=powerFraction  SampleTime=0
  Terminator : Terminator
  Terminator1 : Terminator
  Terminator2 : Terminator
  FRACTIONAL NEUTRON DENSITY : Outport
  wires:
  CORE TEMPERATURE/1 -> Terminator/1
  "XeCore, [cm^2]"/1 -> Terminator1/1
  FlowFrac/1 -> Terminator2/1
  Product/1 -> FRACTIONAL NEUTRON DENSITY/1
  Step/1 -> Product/1
  From Workspace/1 -> Product/2

== system MSDRPrimaryLoop_LoadFollow/Reactor/Reactivity&PKE/Reactivity&PKE ==
  FlowFrac : Inport
  CORE TEMPERATURE : Inport  Port=2
  "XeCore, [cm^2]" : Inport  Port=3
  PKE SOLVER : Subsystem
  REACTIVITY : Subsystem
      settings: PortSchema="{\"entries\":[{\"content\":{\"sides\":[{\"content\":{\"connectorIds\":[\"In1\",\"In2\"]},\"type\":\"ConnectorPlacement.EquallySpacedRectSide\",\"uuid\":\"26ed18f9-521e-467a-8165-f91acdea59eb\"},{\"content\":{\"connectorIds\":[\"Out1\"],\"side\":\"RIGHT\"},\"type\":\"ConnectorPlacement.EquallySpacedRectSide\",\"uuid\":\"cdbabf16-95d7-4a8a-8589-d756110a110a\"},{\"content\":{\"connectorIds\":[],\"side\":\"TOP\"},\"type\":\"ConnectorPlacement.EquallySpacedRectSide\",\"uuid\":\"d0e29e64-a56b-43ad-b460-16ed8821da85\"},{\"content\":{\"connectorIds\":[\"In3\"],\"side\":\"BOTTOM\"},\"type\":\"ConnectorPlacement.EquallySpacedRectSide\",\"uuid\":\"b0e3ee0c-d165-4d95-a563-1f49b7a55c7b\"}]},\"type\":\"ConnectorPlacement.EquallySpacedConnector\",\"uuid\":\"3367cf9a-8030-444c-bb96-bbcb6f025241\"}],\"packageUris\":[\"http://schema.mathworks.com/mf0/Connector/R2020b\"],\"version\":\"1.0\"}"
  Xe and Sm : Subsystem
  FRACTIONAL NEUTRON DENSITY : Outport
  wires:
  CORE TEMPERATURE/1 -> REACTIVITY/1(CORE TEMPERATURE)
  Xe and Sm/1(Poison Level) -> REACTIVITY/2(Poison Level)
  REACTIVITY/1(TOTAL REACTIVITY FEEDBACK) -> PKE SOLVER/1(REACTIVITY FEEDBACK)
  FlowFrac/1 -> PKE SOLVER/2(FLOW FRACTION)
  PKE SOLVER/1(FRACTIONAL NEUTRON DENSITY) -> REACTIVITY/3(P), FRACTIONAL NEUTRON DENSITY/1, Xe and Sm/2(NeutronFraction)
  "XeCore, [cm^2]"/1 -> Xe and Sm/1("XeCore, [cm^2]")

== system MSDRPrimaryLoop_LoadFollow/pipePHXToReactor/XenonCalc/Gas ==
  XeGIn : Inport
  Interphase : Inport  Port=2
  GasRef : Inport  Port=3
  VolumeRate : Inport  Port=4
  Add : Sum  Inputs=+---
  Add1 : Sum  Inputs=+-
  Add2 : Sum
  Constant : Constant
  Gain2 : Gain  Gain=xeDecayConstant
  Gain4 : Gain  Gain=0.5/Area
  LiquidFlowRate : Product
  LiquidVolume : Product  Inputs=*/
  MixtureVolume : Gain  Gain=1/Volume
  PhaseMass : Integrator  LimitOutput=on  LowerSaturationLimit=0
  Subsystem : Subsystem  ReferencedSubsystem=GasToAlpha
  XeGOut : Outport
  GxGas : Outport  Port=2
  wires:
  LiquidFlowRate/1 -> XeGOut/1, Add2/2, Add/3
  Subsystem/1 -> Add1/2
  LiquidVolume/1 -> LiquidFlowRate/2
  Add/1 -> PhaseMass/1
  Constant/1 -> Add1/1
  MixtureVolume/1 -> LiquidVolume/1
  Add1/1 -> LiquidVolume/2
  VolumeRate/1 -> LiquidFlowRate/1
  GasRef/1 -> Subsystem/1
  XeGIn/1 -> Add/1, Add2/1
  Gain2/1 -> Add/4
  PhaseMass/1 -> Gain2/1, MixtureVolume/1
  Gain4/1 -> GxGas/1
  Add2/1 -> Gain4/1
  Interphase/1 -> Add/2

== system MSDRPrimaryLoop_LoadFollow/pipePHXToReactor/XenonCalc/InterphaseTranfser ==
  note: This local to volume isn't strick. Either add an integral or reduce the length of the node if variation is large.
  GxSalt : Inport
  GasRef : Inport  Port=2
  GxGas : Inport  Port=3
  PLoss : Inport  Port=4
  VolumeRate : Inport  Port=5
  Constant : Constant  Value=Dh
  Constitutive : Subsystem
      settings: PortSchema="{\"entries\":[{\"content\":{\"sides\":[{\"content\":{\"connectorIds\":[\"In1\",\"LConn1\",\"In2\",\"In3\",\"In4\"]},\"type\":\"ConnectorPlacement.EquallySpacedRectSide\",\"uuid\":\"b30af6c3-7c55-4661-bc76-939f1c8a4177\"},{\"content\":{\"connectorIds\":[\"Out1\",\"Out2\",\"Out3\",\"Out4\",\"Out5\",\"Out6\",\"Out7\",\"Out8\",\"Out9\"],\"side\":\"RIGHT\"},\"type\":\"ConnectorPlacement.EquallySpacedRectSide\",\"uuid\":\"0b137634-5e01-4bd6-8381-72b0699f5835\"},{\"content\":{\"connectorIds\":[],\"side\":\"TOP\"},\"type\":\"ConnectorPlacement.EquallySpacedRectSide\",\"uuid\":\"06046061-3240-493e-a0a3-282c9541adae\"}]},\"type\":\"ConnectorPlacement.EquallySpacedConnector\",\"uuid\":\"b0591291-fd4b-4355-beaa-e569a19c4b12\"}],\"packageUris\":[\"http://schema.mathworks.com/mf0/Connector/R2020b\"],\"version\":\"1.0\"}"
  MixtureVolume : Gain  Gain=Volume
  String Constant : StringConstant  String="\"downwards\""
  Subsystem : Subsystem  ReferencedSubsystem=kCalculation
      settings: PortSchema="{\"entries\":[{\"content\":{\"sides\":[{\"content\":{\"connectorIds\":[\"In2\",\"In3\",\"In4\",\"In5\",\"In6\",\"In7\",\"In8\",\"In1\"]},\"type\":\"ConnectorPlacement.EquallySpacedRectSide\",\"uuid\":\"002a6616-4b3b-4d3e-9efd-a784f6bbe134\"},{\"content\":{\"connectorIds\":[\"Out1\",\"Out2\"],\"side\":\"RIGHT\"},\"type\":\"ConnectorPlacement.EquallySpacedRectSide\",\"uuid\":\"da6acc14-6515-461b-8149-f4cbf493a4dd\"},{\"content\":{\"connectorIds\":[],\"side\":\"TOP\"},\"type\":\"ConnectorPlacement.EquallySpacedRectSide\",\"uuid\":\"939e49a4-f3cd-4ed3-a7a5-6bbefe0ae08a\"}]},\"type\":\"ConnectorPlacement.EquallySpacedConnector\",\"uuid\":\"8f0c794e-eb76-47c6-abaf-8e07cad1f307\"}],\"packageUris\":[\"http://schema.mathworks.com/mf0/Connector/R2020b\"],\"version\":\"1.0\"}"
  Subsystem1 : Subsystem  ReferencedSubsystem=GasToAlpha
  Transfer Term : MATLAB Function  TreatAsAtomicUnit=on
  Ref : PMIOPort  Side=Left
  TranfserRate : Outport
  wires:
  Transfer Term/1(volRate) -> MixtureVolume/1
  MixtureVolume/1 -> TranfserRate/1
  VolumeRate/1 -> Constitutive/3(VolumeRate)
  GasRef/1 -> Subsystem1/1
  Subsystem1/1 -> Constitutive/1(alpha), Transfer Term/3(alpha)
  Constitutive/1(ul) -> Transfer Term/4(ul)
  Constitutive/2(ug) -> Transfer Term/5(ug)
  Constant/1 -> Subsystem/7, Constitutive/4(Diam)
  GxSalt/1 -> Transfer Term/1(GxS)
  GxGas/1 -> Transfer Term/2(GxG)
  Subsystem/1 -> Transfer Term/7(dsm)
  Subsystem/2 -> Transfer Term/8(k)
  PLoss/1 -> Constitutive/2(PLoss)
  Constitutive/4(Re) -> Subsystem/2
  Constitutive/3(K) -> Transfer Term/6(K)
  Constitutive/5(Sc) -> Subsystem/3
  Constitutive/6(Diff) -> Subsystem/4
  Constitutive/7(alphaC) -> Subsystem/5
  Constitutive/8(dsm) -> Subsystem/6
  Constitutive/9(f_m) -> Subsystem/1
  String Constant/1 -> Subsystem/8
  connections:
  Constitutive/LConn1 -- Ref/RConn1

== system MSDRPrimaryLoop_LoadFollow/pipePHXToReactor/XenonCalc/Salt ==
  XeLIn : Inport  PortDimensions=1
  IodineSNumberDensity : Inport  Port=2  PortDimensions=1
  T_f_ave : Inport  Port=3
  GasRef : Inport  Port=4  PortDimensions=1
  VolumeRate : Inport  Port=5
  Interphase : Inport  Port=6
  Add : Sum  Inputs=+++--  InputSameDT=on
  Add1 : Sum
  Decay : Gain  Gain=xeDecayConstant
  Gain1 : Gain  Gain=0.5/Area
  InPipeGeneration : Subsystem
      settings: PortSchema="{\"entries\":[{\"content\":{\"sides\":[{\"content\":{\"connectorIds\":[\"In1\"]},\"type\":\"ConnectorPlacement.EquallySpacedRectSide\",\"uuid\":\"cf58f9e2-4051-4ec0-bfd5-a375f3464f67\"},{\"content\":{\"connectorIds\":[\"Out1\"],\"side\":\"RIGHT\"},\"type\":\"ConnectorPlacement.EquallySpacedRectSide\",\"uuid\":\"cf475b22-0422-4ebc-b148-ab559744c6ba\"},{\"content\":{\"connectorIds\":[],\"side\":\"TOP\"},\"type\":\"ConnectorPlacement.EquallySpacedRectSide\",\"uuid\":\"15cc78ce-ee79-4f49-b098-b77c0b2a8ba1\"},{\"content\":{\"connectorIds\":[\"In2\"],\"side\":\"BOTTOM\"},\"type\":\"ConnectorPlacement.EquallySpacedRectSide\",\"uuid\":\"64f5be1f-19d6-4b5f-ac24-c41659a6a539\"}]},\"type\":\"ConnectorPlacement.EquallySpacedConnector\",\"uuid\":\"1fb1607a-ceed-4d70-a511-7b706be0d7ea\"}],\"packageUris\":[\"http://schema.mathworks.com/mf0/Connector/R2020b\"],\"version\":\"1.0\"}"
  LiquidFlowRate : Product
  LiquidVolume : Product  Inputs=*/
  MixtureVolume : Gain  Gain=1/Volume
  PhaseMass : Integrator  LimitOutput=on  LowerSaturationLimit=0
  Subsystem1 : Subsystem
  XeLOut : Outport  PortDimensions=1
  GxSalt : Outport  Port=2
  wires:
  LiquidFlowRate/1 -> Add/5, XeLOut/1, Add1/2
  IodineSNumberDensity/1 -> InPipeGeneration/1(IodineSNumberDensity)
  LiquidVolume/1 -> LiquidFlowRate/2
  Add/1 -> PhaseMass/1
  MixtureVolume/1 -> LiquidVolume/1
  VolumeRate/1 -> LiquidFlowRate/1
  T_f_ave/1 -> InPipeGeneration/2(T_f_ave)
  PhaseMass/1 -> Decay/1, MixtureVolume/1
  GasRef/1 -> Subsystem1/1(Gas)
  Subsystem1/1(1-alpha) -> LiquidVolume/2
  InPipeGeneration/1("XenonGenerationRate, [kg/s]") -> Add/2
  XeLIn/1 -> Add1/1, Add/1
  Add1/1 -> Gain1/1
  Gain1/1 -> GxSalt/1
  Interphase/1 -> Add/3
  Decay/1 -> Add/4

== system MSDRPrimaryLoop_LoadFollow/pipePumpToPHX/XenonCalc/Gas ==
  XeGIn : Inport
  Interphase : Inport  Port=2
  GasRef : Inport  Port=3
  VolumeRate : Inport  Port=4
  Add : Sum  Inputs=+---
  Add1 : Sum  Inputs=+-
  Add2 : Sum
  Constant : Constant
  Gain2 : Gain  Gain=xeDecayConstant
  Gain4 : Gain  Gain=0.5/Area
  LiquidFlowRate : Product
  LiquidVolume : Product  Inputs=*/
  MixtureVolume : Gain  Gain=1/Volume
  PhaseMass : Integrator  LimitOutput=on  LowerSaturationLimit=0
  Subsystem : Subsystem  ReferencedSubsystem=GasToAlpha
  XeGOut : Outport
  GxGas : Outport  Port=2
  wires:
  LiquidFlowRate/1 -> XeGOut/1, Add2/2, Add/3
  Subsystem/1 -> Add1/2
  LiquidVolume/1 -> LiquidFlowRate/2
  Add/1 -> PhaseMass/1
  Constant/1 -> Add1/1
  MixtureVolume/1 -> LiquidVolume/1
  Add1/1 -> LiquidVolume/2
  VolumeRate/1 -> LiquidFlowRate/1
  GasRef/1 -> Subsystem/1
  XeGIn/1 -> Add/1, Add2/1
  Gain2/1 -> Add/4
  PhaseMass/1 -> Gain2/1, MixtureVolume/1
  Gain4/1 -> GxGas/1
  Add2/1 -> Gain4/1
  Interphase/1 -> Add/2

== system MSDRPrimaryLoop_LoadFollow/pipePumpToPHX/XenonCalc/InterphaseTranfser ==
  note: This local to volume isn't strick. Either add an integral or reduce the length of the node if variation is large.
  GxSalt : Inport
  GasRef : Inport  Port=2
  GxGas : Inport  Port=3
  PLoss : Inport  Port=4
  VolumeRate : Inport  Port=5
  Constant : Constant  Value=Dh
  Constitutive : Subsystem
      settings: PortSchema="{\"entries\":[{\"content\":{\"sides\":[{\"content\":{\"connectorIds\":[\"In1\",\"LConn1\",\"In2\",\"In3\",\"In4\"]},\"type\":\"ConnectorPlacement.EquallySpacedRectSide\",\"uuid\":\"b30af6c3-7c55-4661-bc76-939f1c8a4177\"},{\"content\":{\"connectorIds\":[\"Out1\",\"Out2\",\"Out3\",\"Out4\",\"Out5\",\"Out6\",\"Out7\",\"Out8\",\"Out9\"],\"side\":\"RIGHT\"},\"type\":\"ConnectorPlacement.EquallySpacedRectSide\",\"uuid\":\"0b137634-5e01-4bd6-8381-72b0699f5835\"},{\"content\":{\"connectorIds\":[],\"side\":\"TOP\"},\"type\":\"ConnectorPlacement.EquallySpacedRectSide\",\"uuid\":\"06046061-3240-493e-a0a3-282c9541adae\"}]},\"type\":\"ConnectorPlacement.EquallySpacedConnector\",\"uuid\":\"b0591291-fd4b-4355-beaa-e569a19c4b12\"}],\"packageUris\":[\"http://schema.mathworks.com/mf0/Connector/R2020b\"],\"version\":\"1.0\"}"
  MixtureVolume : Gain  Gain=Volume
  String Constant : StringConstant  String="\"horizontal\""
  Subsystem : Subsystem  ReferencedSubsystem=kCalculation
      settings: PortSchema="{\"entries\":[{\"content\":{\"sides\":[{\"content\":{\"connectorIds\":[\"In2\",\"In3\",\"In4\",\"In5\",\"In6\",\"In7\",\"In8\",\"In1\"]},\"type\":\"ConnectorPlacement.EquallySpacedRectSide\",\"uuid\":\"002a6616-4b3b-4d3e-9efd-a784f6bbe134\"},{\"content\":{\"connectorIds\":[\"Out1\",\"Out2\"],\"side\":\"RIGHT\"},\"type\":\"ConnectorPlacement.EquallySpacedRectSide\",\"uuid\":\"da6acc14-6515-461b-8149-f4cbf493a4dd\"},{\"content\":{\"connectorIds\":[],\"side\":\"TOP\"},\"type\":\"ConnectorPlacement.EquallySpacedRectSide\",\"uuid\":\"939e49a4-f3cd-4ed3-a7a5-6bbefe0ae08a\"}]},\"type\":\"ConnectorPlacement.EquallySpacedConnector\",\"uuid\":\"8f0c794e-eb76-47c6-abaf-8e07cad1f307\"}],\"packageUris\":[\"http://schema.mathworks.com/mf0/Connector/R2020b\"],\"version\":\"1.0\"}"
  Subsystem1 : Subsystem  ReferencedSubsystem=GasToAlpha
  Transfer Term : MATLAB Function  TreatAsAtomicUnit=on
  Ref : PMIOPort  Side=Left
  TranfserRate : Outport
  wires:
  Transfer Term/1(volRate) -> MixtureVolume/1
  MixtureVolume/1 -> TranfserRate/1
  VolumeRate/1 -> Constitutive/3(VolumeRate)
  GasRef/1 -> Subsystem1/1
  Subsystem1/1 -> Constitutive/1(alpha), Transfer Term/3(alpha)
  Constitutive/1(ul) -> Transfer Term/4(ul)
  Constitutive/2(ug) -> Transfer Term/5(ug)
  Constant/1 -> Subsystem/7, Constitutive/4(Diam)
  GxSalt/1 -> Transfer Term/1(GxS)
  GxGas/1 -> Transfer Term/2(GxG)
  Subsystem/1 -> Transfer Term/7(dsm)
  Subsystem/2 -> Transfer Term/8(k)
  PLoss/1 -> Constitutive/2(PLoss)
  Constitutive/4(Re) -> Subsystem/2
  Constitutive/3(K) -> Transfer Term/6(K)
  Constitutive/5(Sc) -> Subsystem/3
  Constitutive/6(Diff) -> Subsystem/4
  Constitutive/7(alphaC) -> Subsystem/5
  Constitutive/8(dsm) -> Subsystem/6
  Constitutive/9(f_m) -> Subsystem/1
  String Constant/1 -> Subsystem/8
  connections:
  Constitutive/LConn1 -- Ref/RConn1

== system MSDRPrimaryLoop_LoadFollow/pipePumpToPHX/XenonCalc/Salt ==
  XeLIn : Inport  PortDimensions=1
  IodineSNumberDensity : Inport  Port=2  PortDimensions=1
  T_f_ave : Inport  Port=3
  GasRef : Inport  Port=4  PortDimensions=1
  VolumeRate : Inport  Port=5
  Interphase : Inport  Port=6
  Add : Sum  Inputs=+++--  InputSameDT=on
  Add1 : Sum
  Decay : Gain  Gain=xeDecayConstant
  Gain1 : Gain  Gain=0.5/Area
  InPipeGeneration : Subsystem
      settings: PortSchema="{\"entries\":[{\"content\":{\"sides\":[{\"content\":{\"connectorIds\":[\"In1\"]},\"type\":\"ConnectorPlacement.EquallySpacedRectSide\",\"uuid\":\"cf58f9e2-4051-4ec0-bfd5-a375f3464f67\"},{\"content\":{\"connectorIds\":[\"Out1\"],\"side\":\"RIGHT\"},\"type\":\"ConnectorPlacement.EquallySpacedRectSide\",\"uuid\":\"cf475b22-0422-4ebc-b148-ab559744c6ba\"},{\"content\":{\"connectorIds\":[],\"side\":\"TOP\"},\"type\":\"ConnectorPlacement.EquallySpacedRectSide\",\"uuid\":\"15cc78ce-ee79-4f49-b098-b77c0b2a8ba1\"},{\"content\":{\"connectorIds\":[\"In2\"],\"side\":\"BOTTOM\"},\"type\":\"ConnectorPlacement.EquallySpacedRectSide\",\"uuid\":\"64f5be1f-19d6-4b5f-ac24-c41659a6a539\"}]},\"type\":\"ConnectorPlacement.EquallySpacedConnector\",\"uuid\":\"1fb1607a-ceed-4d70-a511-7b706be0d7ea\"}],\"packageUris\":[\"http://schema.mathworks.com/mf0/Connector/R2020b\"],\"version\":\"1.0\"}"
  LiquidFlowRate : Product
  LiquidVolume : Product  Inputs=*/
  MixtureVolume : Gain  Gain=1/Volume
  PhaseMass : Integrator  LimitOutput=on  LowerSaturationLimit=0
  Subsystem1 : Subsystem
  XeLOut : Outport  PortDimensions=1
  GxSalt : Outport  Port=2
  wires:
  LiquidFlowRate/1 -> Add/5, XeLOut/1, Add1/2
  IodineSNumberDensity/1 -> InPipeGeneration/1(IodineSNumberDensity)
  LiquidVolume/1 -> LiquidFlowRate/2
  Add/1 -> PhaseMass/1
  MixtureVolume/1 -> LiquidVolume/1
  VolumeRate/1 -> LiquidFlowRate/1
  T_f_ave/1 -> InPipeGeneration/2(T_f_ave)
  PhaseMass/1 -> Decay/1, MixtureVolume/1
  GasRef/1 -> Subsystem1/1(Gas)
  Subsystem1/1(1-alpha) -> LiquidVolume/2
  InPipeGeneration/1("XenonGenerationRate, [kg/s]") -> Add/2
  XeLIn/1 -> Add1/1, Add/1
  Add1/1 -> Gain1/1
  Gain1/1 -> GxSalt/1
  Interphase/1 -> Add/3
  Decay/1 -> Add/4
